simulink model "ModeltheMavic_close_loop_attitude"  (R2018b)
settings: Solver=VariableStepAuto  StartTime=0.0  StopTime=100  RelTol=1e-3
libraries: simulink x1
settings Model: Creator=cnit355  LastModifiedBy=cnit355

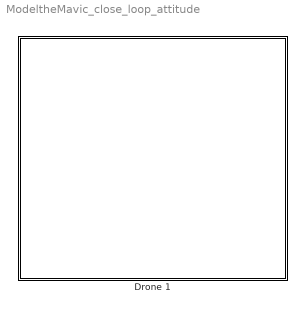
== system ModeltheMavic_close_loop_attitude ==
  Drone 1 : Subsystem  Tag=Drone 1

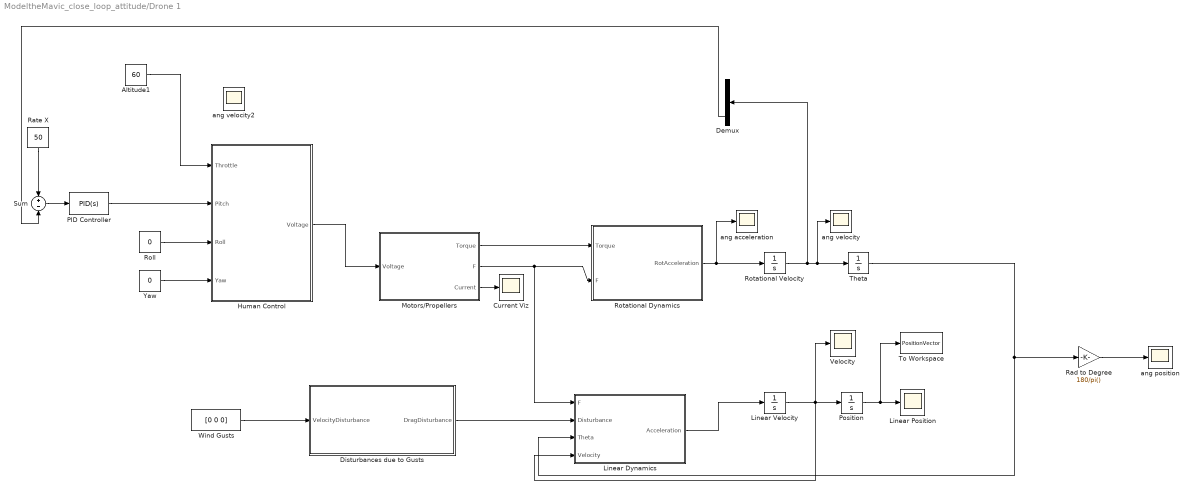
== system ModeltheMavic_close_loop_attitude/Drone 1 ==
  Altitude1 : Constant  Value=60
  Current Viz : Scope
  Demux : Demux  Outputs=3
  Disturbances due to Gusts : MATLAB Function  TreatAsAtomicUnit=on
  Human Control : MATLAB Function  TreatAsAtomicUnit=on
  Linear Dynamics : MATLAB Function  TreatAsAtomicUnit=on
  Linear Position : Scope
  Linear Velocity : Integrator
  Motors/Propellers : MATLAB Function  TreatAsAtomicUnit=on
  PID Controller : simulink/Continuous/PID Controller  Controller=PID  Form=Parallel  TimeDomain=Continuous-time  SampleTime=-1  IntegratorMethod=Forward Euler  FilterMethod=Forward Euler  ControllerParametersSource=internal  P=-202.816  I=-391.556  D=5.561  UseFilter=on  N=100  TunerSelectOption=Transfer Function Based (PID Tuner App)  InitialConditionSource=internal  InitialConditionForIntegrator=0  InitialConditionForFilter=0  DifferentiatorICPrevScaledInput=0  ExternalReset=none  TrackingMode=off  Kt=1  LimitOutput=on  UpperSaturationLimit=100  LowerSaturationLimit=0  LinearizeAsGain=on  AntiWindupMode=clamping  Kb=1  POutMin=[]  POutMax=[]  IOutMin=[]  IOutMax=[]  DOutMin=[]  DOutMax=[]  NOutMin=[]  NOutMax=[]  SumOutMin=[]  SumOutMax=[]  SaturationOutMin=[]  SaturationOutMax=[]  PParamMin=[]  PParamMax=[]  IParamMin=[]  IParamMax=[]  DParamMin=[]  DParamMax=[]  NParamMin=[]  NParamMax=[]  KbParamMin=[]  KbParamMax=[]  KtParamMin=[]  KtParamMax=[]  KbOutMin=[]  KbOutMax=[]  KtOutMin=[]  KtOutMax=[]  IntegratorOutMin=[]  IntegratorOutMax=[]  FilterOutMin=[]  FilterOutMax=[]  SumI1OutMin=[]  SumI1OutMax=[]  SumI2OutMin=[]  SumI2OutMax=[]  SumI3OutMin=[]  SumI3OutMax=[]  SumI4OutMin=[]  SumI4OutMax=[]  SumDOutMin=[]  SumDOutMax=[]  DifferentiatorOutMin=[]  DifferentiatorOutMax=[]  FilterDiffOutCoefMin=[]  FilterDiffOutCoefMax=[]  ReciprocalOutMin=[]  ReciprocalOutMax=[]  SumDenOutMin=[]  SumDenOutMax=[]  SumNumOutMin=[]  SumNumOutMax=[]  DivideOutMin=[]  DivideOutMax=[]  IntegratorContinuousStateAttributes=''  IntegratorStateMustResolveToSignalObject=off  IntegratorRTWStateStorageClass=Auto  FilterContinuousStateAttributes=''  FilterStateMustResolveToSignalObject=off  FilterRTWStateStorageClass=Auto  ParallelPVariant=InternalParameters  IdealPVariant=Disabled  IVariant=InternalParameters  DVariant=InternalParameters  IntegratorVariant=Continuous  SatVariant=Enabled  AWVariant=ContClampingParallel  PCopyVariant=Disabled  TRVariant=Disabled  FdbkBlocksVariant=Forward  IdealPFdbkVariant=Disabled  SatFdbkVariant=Disabled  DerivativeFilterVariant=ContFilter  NVariant=InternalParameters  NCopyVariant=Disabled  FilterICVariant=InternalICsFilter  IntegratorICVariant=InternalICs  ExternalResetVariant=Disabled  TRSumVariant=Passthrough  SumFdbkVariant=Disabled  SumVariant=Sum_PID
  Position : Integrator
  Rad to Degree : Gain  Gain=180/pi()
  Rate X : Constant  Value=50
  Roll : Constant  Value=0
  Rotational Dynamics : MATLAB Function  TreatAsAtomicUnit=on
  Rotational Velocity : Integrator
  Sum : Sum  Inputs=+-
  Theta : Integrator
  To Workspace : ToWorkspace  VariableName=PositionVector  SampleTime=-1
      settings: Save2DSignal=2-D array (concatenate along first dimension)
  "Velocity " : Scope
  Wind Gusts : Constant  Value=[0 0 0]
  Yaw : Constant  Value=0
  ang acceleration : Scope
  "ang position " : Scope
  ang velocity : Scope
  ang velocity2 : Scope
  wires:
  Theta/1 -> Rad to Degree/1, Linear Dynamics/3(Theta)
  Motors/Propellers/3(Current) -> Current Viz/1
  Rotational Velocity/1 -> Demux/1, ang velocity/1, Theta/1
  Linear Velocity/1 -> "Velocity "/1, Linear Dynamics/4(Velocity), Position/1
  Disturbances due to Gusts/1(DragDisturbance) -> Linear Dynamics/2(Disturbance)
  Rotational Dynamics/1(RotAcceleration) -> ang acceleration/1, Rotational Velocity/1
  Rad to Degree/1 -> "ang position "/1
  Position/1 -> To Workspace/1, Linear Position/1
  Linear Dynamics/1(Acceleration) -> Linear Velocity/1
  Human Control/1(Voltage) -> Motors/Propellers/1(Voltage)
  Yaw/1 -> Human Control/4(Yaw)
  Roll/1 -> Human Control/3(Roll)
  Motors/Propellers/1(Torque) -> Rotational Dynamics/1(Torque)
  Motors/Propellers/2(F) -> Linear Dynamics/1(F), Rotational Dynamics/2(F)
  Wind Gusts/1 -> Disturbances due to Gusts/1(VelocityDisturbance)
  Rate X/1 -> Sum/1
  Demux/3 -> Sum/2
  Sum/1 -> PID Controller/1
  Altitude1/1 -> Human Control/1(Throttle)
  PID Controller/1 -> Human Control/2(Pitch)

== matlab function ModeltheMavic_close_loop_attitude/Drone 1/Rotational Dynamics ==
  data: Torque input; RotAcceleration output; F input
function RotAcceleration = fcn(Torque, F)
Moment = [0 0 0];
RotAcceleration = [0 0 0]; 
I = [0.003, 0.003, 0.007]; %moment of inertia

Moment(1) =  (F(3)+F(4)) * 0.237/2 - (F(1)+F(2))*0.237/2;
Moment(2) =  (F(3)+F(2)) * 0.237/2 - (F(1)+F(4))*0.237/2;
Moment(3) =  Torque(4) - Torque(1) + Torque(2) - Torque(3); %yaw

for i=1:3
    RotAcceleration(i) = Moment(i) / I(i);
end

== matlab function ModeltheMavic_close_loop_attitude/Drone 1/Motors//Propellers ==
  data: Voltage input; Torque output; F output; Current output
function [Torque, F, Current] = fcn(Voltage)

RPM = [0 0 0 0];
Torque = [0 0 0 0];
Current = [0 0 0 0];
F = [0 0 0 0];

for i=1:4
    RPM(i) = -2.6931*Voltage(i)^3+1400*Voltage(i);
    Ct = 2 * 10 ^-15 * RPM(i)^3-4*10^-11*RPM(i)^2+3*10^-7*RPM(i)+0.1013;
    F(i) = Ct * 1.225*(RPM(i)/60)^2 * 0.2^4;%0.2 = diameter of propeller
    Torque(i) = 4*10^-14*RPM(i)^3+8*10^-12*RPM(i)^2+3*10^-6*RPM(i);
    Current(i) = 1400*Torque(i);
end

== matlab function ModeltheMavic_close_loop_attitude/Drone 1/Linear Dynamics ==
  data: F input; Acceleration output; Disturbance input; Theta input; Velocity input
function Acceleration  = fcn(F,Disturbance,Theta,Velocity)
m=0.743;
g=9.81;
A=[0.0197 0.0197 0.0512];
rho=1.225;
Cd=1;

Acceleration=[0 0 0];
Force=[0 0 0];
Fprop=[0;0;0];

Fprop(1,1)=sin(Theta(2))*cos(Theta(1))*(F(1)+F(2)+F(3)+F(4));
Fprop(2,1)=sin(Theta(1))*cos(Theta(2))*(F(1)+F(2)+F(3)+F(4));

Fprop(3,1)=(F(1)+F(2)+F(3)+F(4))*cos(Theta(1))*cos(Theta(2));

ThetaXY = -atan2(Fprop(1),Fprop(2));
XY2D=sqrt(Fprop(1)^2+Fprop(2)^2);
if Fprop(3)>=0
    Fprop(1)=XY2D*sin(Theta(3)+ThetaXY);
    Fprop(2)=XY2D*cos(Theta(3)+ThetaXY);
else
     Fprop(1)=XY2D*sin(-Theta(3)+ThetaXY);
    Fprop(2)=XY2D*cos(-Theta(3)+ThetaXY);
end
    
if Velocity(1)<0
Force(1)=Fprop(1)-Disturbance(1)+0.5*rho*Velocity(1)^2*A(1)*Cd;
else 
    Force(1)=Fprop(1)-Disturbance(1)-0.5*rho*Velocity(1)^2*A(1)*Cd;
end

if Velocity(2)<0
Force(2)=Fprop(2)-Disturbance(2)+0.5*rho*Velocity(2)^2*A(2)*Cd;
else 
    Force(2)=Fprop(2)-Disturbance(2)-0.5*rho*Velocity(2)^2*A(2)*Cd;
end

if Velocity(3)<0
Force(3)=Fprop(3)+0.5*rho*Velocity(3)^2*A(3)*Cd-m*g-Disturbance(3);
else 
Force(3)=Fprop(3)-0.5*rho*Velocity(3)^2*A(3)*Cd-m*g-Disturbance(3);
end

for i=1:3
    Acceleration(i)=Force(i)/m;
end

== matlab function ModeltheMavic_close_loop_attitude/Drone 1/Disturbances due to Gusts ==
  data: VelocityDisturbance input; DragDisturbance output
function DragDisturbance = fcn(VelocityDisturbance)
A=[0.0197 0.0197 0.0197*2*1.3]; %x,y,z direction
DragDisturbance=[0 0 0];
rho=1.225; %sea level
Cd=1; %coefficient of drag

for i=1:3
    if VelocityDisturbance(i) < 0
        DragDisturbance(i)= 0.5*rho*VelocityDisturbance(i)^2*A(i)*Cd;
    else
        DragDisturbance(i)= -0.5*rho*VelocityDisturbance(i)^2*A(i)*Cd;
    end
end

== matlab function ModeltheMavic_close_loop_attitude/Drone 1/Human Control ==
  data: Throttle input; Voltage output; Pitch input; Roll input; Yaw input
function Voltage = fcn(Throttle, Pitch, Roll, Yaw)

Correct = 0; %correction of final voltage

%condition of each input 
%Throttle <- increase and decrease pitch roll yaw symetrically

if (Pitch/2+Roll/2+Yaw/2) > (100-Throttle) % -50 ~ +50
   
    Correct = ((Pitch/2 + Roll/2 + Yaw/2) - (100 - Throttle));
       
end

if (Pitch/2+Roll/2+Yaw/2) > (Throttle) %Enough space for other size // make it never go down to 10%... -10 will result in false movement

    if Correct < ((Pitch/2 + Roll/2 + Yaw/2) - (Throttle - 10)) % jf too big, take excess
        Correct = ((Pitch/2 + Roll/2 + Yaw/2) - (Throttle - 10)) ;   
    end
            
end

if Correct ~= 0 
    %Correct pitch, roll, yaw from user input
    Pitch = Pitch - Correct / 3 * 2; %distribute excess to pitch, roll, and yaw
    Roll = Roll - Correct / 3 * 2;
    Yaw = Yaw - Correct / 3 * 2;
end

%voltage for each motor
Voltage = [(Throttle - Pitch / 2 - Roll / 2 - Yaw / 2)*11.4/100%percent=> divide by 100 /  voltage max = 11.4
    (Throttle - Pitch / 2 + Roll / 2 + Yaw / 2)*11.4/100
    (Throttle + Pitch / 2 + Roll / 2 - Yaw / 2)*11.4/100
    (Throttle + Pitch / 2 - Roll / 2 + Yaw / 2)*11.4/100]
